simulink model "PruebaN5"  (R2024b)
settings: Solver=ode45  StartTime=0.0  StopTime=10  RelTol=1e-3
values from neighbouring files (symbols this model uses):
  T = 10e-3    (= 0.01)    [Proceso.m]    (also in regdiagSISOsep.m = Reg.Ts; regdiagsep.m = Reg.Ts; regsep.m = Reg.Ts)
undefined symbols (not defined in the file or in its folder): N, nl, nr, RegBal_Len2_ext, RegBal_Len3_ext, RegBal_Len4_ext, RegBal_Len5_ext, RegDiag_Len2_ext, RegDiag_Len3_ext, RegDiag_Len4_ext, RegDiag_Len5_ext, SR_Bal
libraries: cstblocks x18
settings Model: Creator=Guillem  LastModifiedBy=jroigro
settings SolverCC: AlgebraicLoopSolver=TrustRegion
settings DataIOCC: LimitDataPoints=on  SaveFormat=Array  SignalLoggingSaveFormat=ModelDataLogs  ReturnWorkspaceOutputs=off
settings OptimizationCC: BlockReduction=off  BooleanDataType=off  LifeSpan=inf
settings DebuggingCC: SaveWithParameterizedLinksMsg=none  UnderspecifiedInitializationDetection=Classic  MergeDetectMultiDrivingBlocksExec=none  SignalResolutionControl=TryResolveAllWithWarning  MultiTaskDSMMsg=warning  MultiTaskCondExecSysMsg=none  UnconnectedInputMsg=warning  UnconnectedOutputMsg=warning  UnconnectedLineMsg=warning  SFUnexpectedBacktrackingDiag=warning  SFNoUnconditionalDefaultTransitionDiag=warning  SFExecutionAtInitializationDiag=none  ArithmeticOperatorsInVariantConditions=warning
settings HardwareCC: ProdBitPerPointer=32  ProdBitPerSizeT=32  ProdBitPerPtrDiffT=32  ProdLargestAtomicFloat=None  ProdIntDivRoundTo=Undefined  ProdEndianess=Unspecified  ProdWordSize=32  ProdHWDeviceType=32-bit Generic  TargetUnknown=on
settings ModelReferenceCC: PropagateSignalLabelsOutOfModel=off
settings SFSimCC: SimUseLocalCustomCode=off  CustomCodeUndefinedFunction=UseInterfaceOnly
settings RTWCC: RTWUseLocalCustomCode=off  GPUComputeCapability=3.5
settings CodeAppCC: StateflowObjectComments=on
settings GRTTargetCC: TargetLangStandard=C89/C90 (ANSI)
settings ConfigComp: CovMetricSettings=dw  CovSaveCumulativeToWorkspaceVar=on  CovSaveSingleToWorkspaceVar=on  CovExternalEMLEnable=off

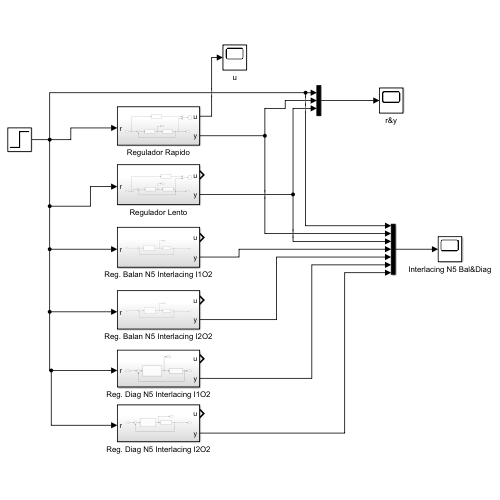
[thumbnail: Simulink's stored preview of the top-level diagram]
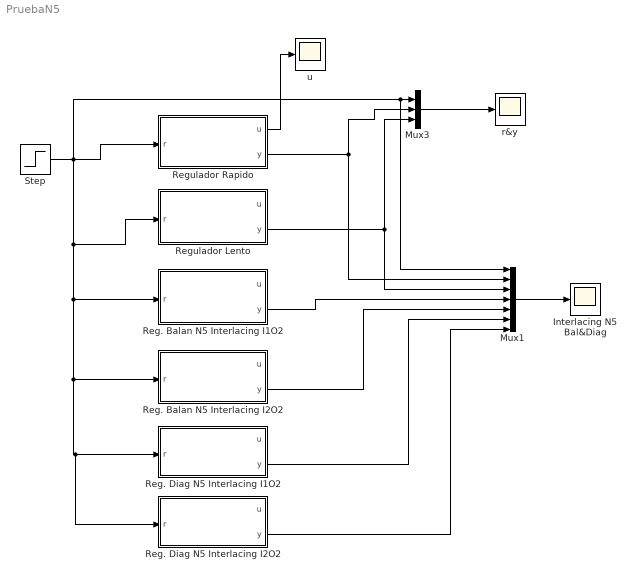
== system PruebaN5 ==
  Interlacing N5 Bal&Diag : Scope
  Mux1 : Mux  Inputs=7
  Mux3 : Mux  Inputs=3
  Reg. Balan N5 Interlacing I1O2 : Subsystem
  Reg. Balan N5 Interlacing I2O2 : Subsystem
  Reg. Diag N5 Interlacing I1O2 : Subsystem
  Reg. Diag N5 Interlacing I2O2 : Subsystem
  Regulador Lento : Subsystem
  Regulador Rapido : Subsystem
  Step : Step  Time=10  Before=1  After=2  SampleTime=0
  r&y : Scope
  u : Scope
  wires:
  Mux3/1 -> r&y/1
  Regulador Rapido/2(y) -> Mux1/2, Mux3/2
  Regulador Rapido/1(u) -> u/1
  Reg. Balan N5 Interlacing I2O2/2(y) -> Mux1/5
  Mux1/1 -> Interlacing N5 Bal&Diag/1
  Regulador Lento/2(y) -> Mux1/3, Mux3/3
  Reg. Balan N5 Interlacing I1O2/2(y) -> Mux1/4
  Step/1 -> Reg. Diag N5 Interlacing I2O2/1(r), Reg. Diag N5 Interlacing I1O2/1(r), Reg. Balan N5 Interlacing I2O2/1(r), Reg. Balan N5 Interlacing I1O2/1(r), Regulador Lento/1(r), Mux1/1, Mux3/1, Regulador Rapido/1(r)
  Reg. Diag N5 Interlacing I1O2/2(y) -> Mux1/6
  Reg. Diag N5 Interlacing I2O2/2(y) -> Mux1/7

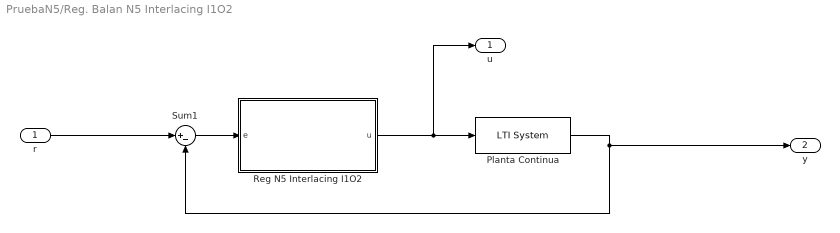
== system PruebaN5/Reg. Balan N5 Interlacing I1O2 ==
  r : Inport
  Planta Continua : cstblocks/LTI System  sys=Planta  IC=[]  PadeOrder=0
  Reg N5 Interlacing I1O2 : Subsystem
  Sum1 : Sum  Inputs=|+-
  u : Outport
  y : Outport  Port=2
  wires:
  Reg N5 Interlacing I1O2/1(u) -> u/1, Planta Continua/1
  Planta Continua/1 -> y/1, Sum1/2
  Sum1/1 -> Reg N5 Interlacing I1O2/1(e)
  r/1 -> Sum1/1

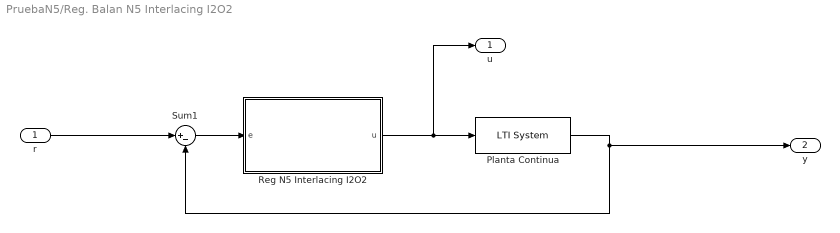
== system PruebaN5/Reg. Balan N5 Interlacing I2O2 ==
  r : Inport
  Planta Continua : cstblocks/LTI System  sys=Planta  IC=[]  PadeOrder=0
  Reg N5 Interlacing I2O2 : Subsystem
  Sum1 : Sum  Inputs=|+-
  u : Outport
  y : Outport  Port=2
  wires:
  r/1 -> Sum1/1
  Reg N5 Interlacing I2O2/1(u) -> u/1, Planta Continua/1
  Sum1/1 -> Reg N5 Interlacing I2O2/1(e)
  Planta Continua/1 -> y/1, Sum1/2

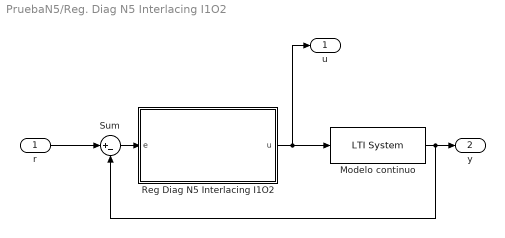
== system PruebaN5/Reg. Diag N5 Interlacing I1O2 ==
  r : Inport
  Modelo continuo : cstblocks/LTI System  sys=Planta  IC=[]  PadeOrder=0
  Reg Diag N5 Interlacing I1O2 : Subsystem
  Sum : Sum  Inputs=|+-
  u : Outport
  y : Outport  Port=2
  wires:
  Reg Diag N5 Interlacing I1O2/1(u) -> Modelo continuo/1, u/1
  r/1 -> Sum/1
  Sum/1 -> Reg Diag N5 Interlacing I1O2/1(e)
  Modelo continuo/1 -> Sum/2, y/1

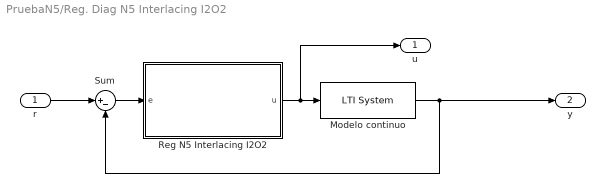
== system PruebaN5/Reg. Diag N5 Interlacing I2O2 ==
  r : Inport
  Modelo continuo : cstblocks/LTI System  sys=Planta  IC=[]  PadeOrder=0
  Reg N5 Interlacing I2O2 : Subsystem
  Sum : Sum  Inputs=|+-
  u : Outport
  y : Outport  Port=2
  wires:
  Modelo continuo/1 -> Sum/2, y/1
  Reg N5 Interlacing I2O2/1(u) -> Modelo continuo/1, u/1
  r/1 -> Sum/1
  Sum/1 -> Reg N5 Interlacing I2O2/1(e)

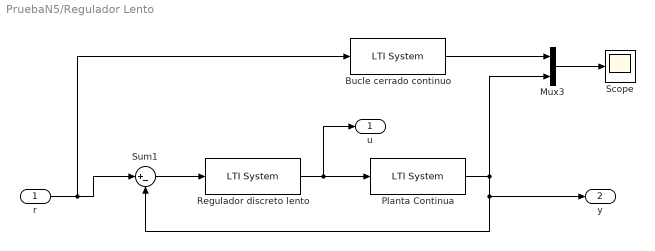
== system PruebaN5/Regulador Lento ==
  r : Inport
  Bucle cerrado continuo : cstblocks/LTI System  sys=BC2  IC=[]  PadeOrder=0
  Mux3 : Mux  Inputs=2
  Planta Continua : cstblocks/LTI System  sys=Planta  IC=[]  PadeOrder=0
  Regulador discreto lento : cstblocks/LTI System  sys=GrN5  IC=[]  PadeOrder=0
  Scope : Scope
  Sum1 : Sum  Inputs=|+-
  u : Outport
  y : Outport  Port=2
  wires:
  r/1 -> Bucle cerrado continuo/1, Sum1/1
  Regulador discreto lento/1 -> u/1, Planta Continua/1
  Sum1/1 -> Regulador discreto lento/1
  Planta Continua/1 -> Sum1/2, y/1, Mux3/2
  Mux3/1 -> Scope/1
  Bucle cerrado continuo/1 -> Mux3/1

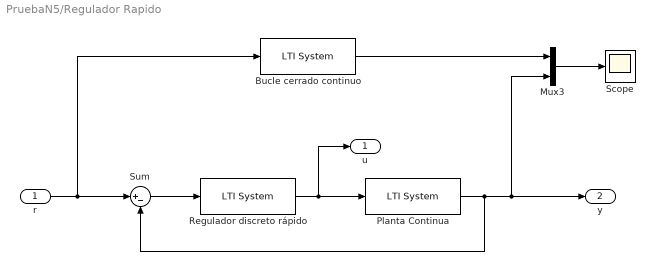
== system PruebaN5/Regulador Rapido ==
  r : Inport
  Bucle cerrado continuo : cstblocks/LTI System  sys=BC1  IC=[]  PadeOrder=0
  Mux3 : Mux  Inputs=2
  Planta Continua : cstblocks/LTI System  sys=Planta  IC=[]  PadeOrder=0
  Regulador discreto rápido : cstblocks/LTI System  sys=Gr  IC=[]  PadeOrder=0
  Scope : Scope
  Sum : Sum  Inputs=|+-
  u : Outport
  y : Outport  Port=2
  wires:
  Regulador discreto rápido/1 -> u/1, Planta Continua/1
  Bucle cerrado continuo/1 -> Mux3/1
  Mux3/1 -> Scope/1
  Sum/1 -> Regulador discreto rápido/1
  Planta Continua/1 -> Mux3/2, y/1, Sum/2
  r/1 -> Sum/1, Bucle cerrado continuo/1

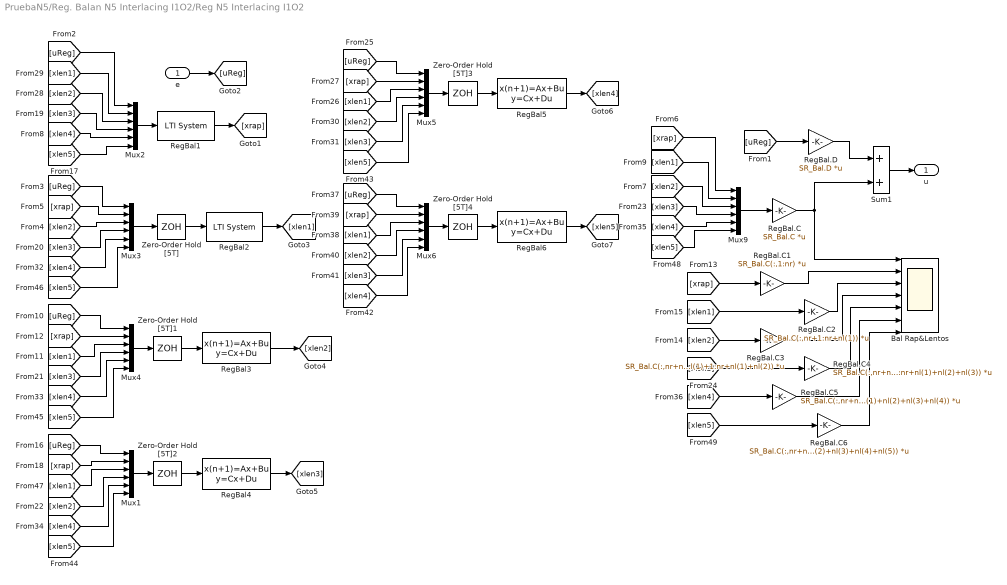
== system PruebaN5/Reg. Balan N5 Interlacing I1O2/Reg N5 Interlacing I1O2 ==
  e : Inport
  Bal Rap&Lentos : Scope  NumInputPorts=7
  Mux{1..6,9} (7 alike) : Mux  Inputs=6
  RegBal.C : Gain  Gain=SR_Bal.C  Multiplication=Matrix(K*u)
  RegBal.C1 : Gain  Gain=SR_Bal.C(:,1:nr)  Multiplication=Matrix(K*u)
  RegBal.C2 : Gain  Gain=SR_Bal.C(:,nr+1:nr+nl(1))  Multiplication=Matrix(K*u)
  RegBal.C3 : Gain  Gain=SR_Bal.C(:,nr+nl(1)+1:nr+nl(1)+nl(2))  Multiplication=Matrix(K*u)
  RegBal.C4 : Gain  Gain=SR_Bal.C(:,nr+nl(1)+nl(2)+1:nr+nl(1)+nl(2)+nl(3))  Multiplication=Matrix(K*u)
  RegBal.C5 : Gain  Gain=SR_Bal.C(:,nr+nl(1)+nl(2)+nl(3)+1:nr+nl(1)+nl(2)+nl(3)+nl(4))  Multiplication=Matrix(K*u)
  RegBal.C6 : Gain  Gain=SR_Bal.C(:,nr+nl(1)+nl(2)+nl(3)+nl(4)+1:nr+nl(1)+nl(2)+nl(3)+nl(4)+nl(5))  Multiplication=Matrix(K*u)
  RegBal.D : Gain  Gain=SR_Bal.D  Multiplication=Matrix(K*u)
  RegBal1 : cstblocks/LTI System  sys=RegBal_Rap  IC=[]  PadeOrder=0
  RegBal2 : cstblocks/LTI System  sys=RegBal_Len1_ext  IC=[]  PadeOrder=0
  RegBal3 : DiscreteStateSpace  A=RegBal_Len2_ext.A  B=RegBal_Len2_ext.B  C=RegBal_Len2_ext.C  D=RegBal_Len2_ext.D  SampleTime=[N*T,T]
  RegBal4 : DiscreteStateSpace  A=RegBal_Len3_ext.A  B=RegBal_Len3_ext.B  C=RegBal_Len3_ext.C  D=RegBal_Len3_ext.D  SampleTime=[N*T,2*T]
  RegBal5 : DiscreteStateSpace  A=RegBal_Len4_ext.A  B=RegBal_Len4_ext.B  C=RegBal_Len4_ext.C  D=RegBal_Len4_ext.D  SampleTime=[N*T,3*T]
  RegBal6 : DiscreteStateSpace  A=RegBal_Len5_ext.A  B=RegBal_Len5_ext.B  C=RegBal_Len5_ext.C  D=RegBal_Len5_ext.D  SampleTime=[N*T,4*T]
  Sum1 : Sum
  Zero-Order Hold [5T]{,1..4} (5 alike) : ZeroOrderHold  SampleTime=[N*T]
  u : Outport
  wires:
  RegBal.D/1 -> Sum1/1
  Mux4/1 -> Zero-Order Hold [5T]1/1
  Mux9/1 -> RegBal.C/1
  Sum1/1 -> u/1
  Mux2/1 -> RegBal1/1
  Mux3/1 -> Zero-Order Hold [5T]/1
  e/1 -> [uReg]
  RegBal.C3/1 -> Bal Rap&Lentos/4
  RegBal.C/1 -> Bal Rap&Lentos/1, Sum1/2
  RegBal.C2/1 -> Bal Rap&Lentos/3
  RegBal2/1 -> [xlen1]
  RegBal.C1/1 -> Bal Rap&Lentos/2
  Zero-Order Hold [5T]/1 -> RegBal2/1
  Zero-Order Hold [5T]1/1 -> RegBal3/1
  RegBal1/1 -> [xrap]
  [uReg] -> RegBal.D/1
  [uReg] -> Mux2/1
  [xlen1] -> Mux2/2
  [xlen2] -> Mux2/3
  [uReg] -> Mux3/1
  [xlen2] -> Mux3/3
  [xrap] -> Mux3/2
  [xrap] -> Mux9/1
  [xlen1] -> Mux9/2
  [xlen2] -> Mux9/3
  RegBal3/1 -> [xlen2]
  [xrap] -> Mux4/2
  [xlen1] -> Mux4/3
  [uReg] -> Mux4/1
  [xlen2] -> RegBal.C3/1
  [xlen1] -> RegBal.C2/1
  [xrap] -> RegBal.C1/1
  [uReg] -> Mux1/1
  [xrap] -> Mux1/2
  RegBal4/1 -> [xlen3]
  Zero-Order Hold [5T]2/1 -> RegBal4/1
  Mux1/1 -> Zero-Order Hold [5T]2/1
  [xlen3] -> Mux2/4
  [xlen3] -> Mux3/4
  [xlen3] -> Mux4/4
  [xlen2] -> Mux1/4
  [xlen3] -> Mux9/4
  [xlen3] -> RegBal.C4/1
  RegBal.C4/1 -> Bal Rap&Lentos/5
  [xlen1] -> Mux5/3
  Zero-Order Hold [5T]3/1 -> RegBal5/1
  [xrap] -> Mux5/2
  [uReg] -> Mux5/1
  Mux5/1 -> Zero-Order Hold [5T]3/1
  [xlen2] -> Mux5/4
  RegBal5/1 -> [xlen4]
  [xlen3] -> Mux5/5
  [xlen4] -> Mux2/5
  [xlen4] -> Mux3/5
  [xlen4] -> Mux4/5
  [xlen4] -> Mux1/5
  [xlen4] -> Mux9/5
  [xlen4] -> RegBal.C5/1
  RegBal.C5/1 -> Bal Rap&Lentos/6
  [xlen3] -> Mux6/5
  RegBal6/1 -> [xlen5]
  [xlen2] -> Mux6/4
  Mux6/1 -> Zero-Order Hold [5T]4/1
  [uReg] -> Mux6/1
  [xrap] -> Mux6/2
  Zero-Order Hold [5T]4/1 -> RegBal6/1
  [xlen1] -> Mux6/3
  [xlen4] -> Mux6/6
  [xlen5] -> Mux5/6
  [xlen5] -> Mux1/6
  [xlen5] -> Mux4/6
  [xlen5] -> Mux3/6
  [xlen1] -> Mux1/3
  [xlen5] -> Mux2/6
  [xlen5] -> Mux9/6
  [xlen5] -> RegBal.C6/1
  RegBal.C6/1 -> Bal Rap&Lentos/7

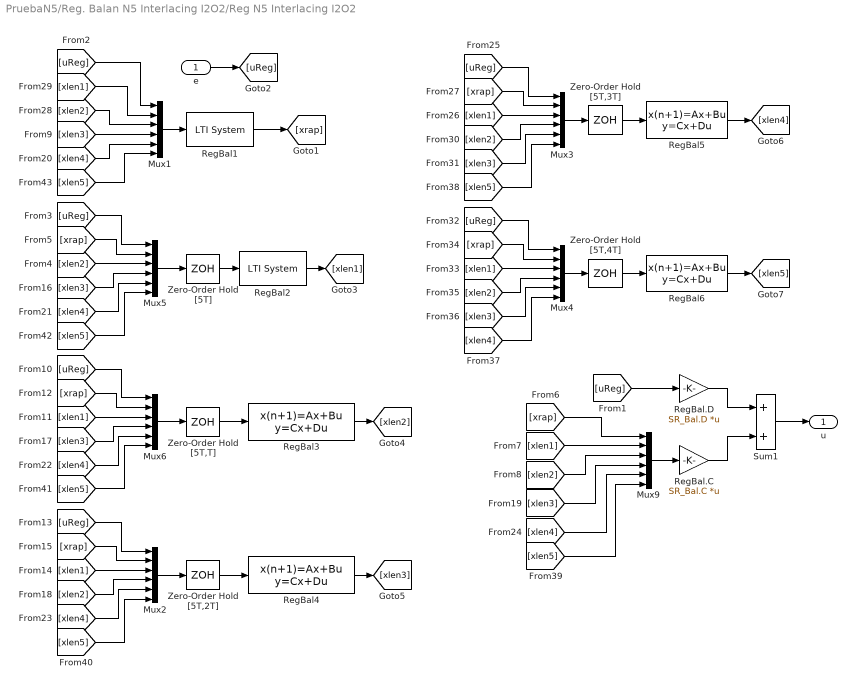
== system PruebaN5/Reg. Balan N5 Interlacing I2O2/Reg N5 Interlacing I2O2 ==
  e : Inport
  Mux{1..6,9} (7 alike) : Mux  Inputs=6
  RegBal.C : Gain  Gain=SR_Bal.C  Multiplication=Matrix(K*u)
  RegBal.D : Gain  Gain=SR_Bal.D  Multiplication=Matrix(K*u)
  RegBal1 : cstblocks/LTI System  sys=RegBal_Rap  IC=[]  PadeOrder=0
  RegBal2 : cstblocks/LTI System  sys=RegBal_Len1_ext  IC=[]  PadeOrder=0
  RegBal3 : DiscreteStateSpace  A=RegBal_Len2_ext.A  B=RegBal_Len2_ext.B  C=RegBal_Len2_ext.C  D=RegBal_Len2_ext.D  SampleTime=[N*T,T]
  RegBal4 : DiscreteStateSpace  A=RegBal_Len3_ext.A  B=RegBal_Len3_ext.B  C=RegBal_Len3_ext.C  D=RegBal_Len3_ext.D  SampleTime=[N*T,2*T]
  RegBal5 : DiscreteStateSpace  A=RegBal_Len4_ext.A  B=RegBal_Len4_ext.B  C=RegBal_Len4_ext.C  D=RegBal_Len4_ext.D  SampleTime=[N*T,3*T]
  RegBal6 : DiscreteStateSpace  A=RegBal_Len5_ext.A  B=RegBal_Len5_ext.B  C=RegBal_Len5_ext.C  D=RegBal_Len5_ext.D  SampleTime=[N*T,4*T]
  Sum1 : Sum
  Zero-Order Hold [5T,2T] : ZeroOrderHold  SampleTime=[N*T,2*T]
  Zero-Order Hold [5T,3T] : ZeroOrderHold  SampleTime=[N*T,3*T]
  Zero-Order Hold [5T,4T] : ZeroOrderHold  SampleTime=[N*T,4*T]
  Zero-Order Hold [5T,T] : ZeroOrderHold  SampleTime=[N*T,T]
  Zero-Order Hold [5T] : ZeroOrderHold  SampleTime=[N*T]
  u : Outport
  wires:
  RegBal.C/1 -> Sum1/2
  Sum1/1 -> u/1
  Mux9/1 -> RegBal.C/1
  Mux6/1 -> Zero-Order Hold [5T,T]/1
  RegBal.D/1 -> Sum1/1
  Zero-Order Hold [5T,T]/1 -> RegBal3/1
  Zero-Order Hold [5T]/1 -> RegBal2/1
  [xlen1] -> Mux1/2
  [xrap] -> Mux5/2
  e/1 -> [uReg]
  Mux5/1 -> Zero-Order Hold [5T]/1
  [xlen2] -> Mux1/3
  [xlen2] -> Mux5/3
  [uReg] -> Mux5/1
  [xrap] -> Mux6/2
  [xlen1] -> Mux6/3
  [uReg] -> Mux6/1
  [uReg] -> Mux1/1
  Mux1/1 -> RegBal1/1
  RegBal1/1 -> [xrap]
  RegBal2/1 -> [xlen1]
  RegBal3/1 -> [xlen2]
  [uReg] -> RegBal.D/1
  [xrap] -> Mux9/1
  [xlen1] -> Mux9/2
  [xlen2] -> Mux9/3
  RegBal4/1 -> [xlen3]
  [uReg] -> Mux2/1
  [xlen1] -> Mux2/3
  [xrap] -> Mux2/2
  Zero-Order Hold [5T,2T]/1 -> RegBal4/1
  Mux2/1 -> Zero-Order Hold [5T,2T]/1
  [xlen3] -> Mux1/4
  [xlen3] -> Mux5/4
  [xlen3] -> Mux6/4
  [xlen2] -> Mux2/4
  [xlen3] -> Mux9/4
  RegBal5/1 -> [xlen4]
  Mux3/1 -> Zero-Order Hold [5T,3T]/1
  [xlen2] -> Mux3/4
  [uReg] -> Mux3/1
  [xrap] -> Mux3/2
  [xlen3] -> Mux3/5
  Zero-Order Hold [5T,3T]/1 -> RegBal5/1
  [xlen1] -> Mux3/3
  [xlen4] -> Mux1/5
  [xlen4] -> Mux5/5
  [xlen4] -> Mux6/5
  [xlen4] -> Mux2/5
  [xlen4] -> Mux9/5
  [uReg] -> Mux4/1
  Zero-Order Hold [5T,4T]/1 -> RegBal6/1
  Mux4/1 -> Zero-Order Hold [5T,4T]/1
  RegBal6/1 -> [xlen5]
  [xlen2] -> Mux4/4
  [xlen3] -> Mux4/5
  [xlen1] -> Mux4/3
  [xrap] -> Mux4/2
  [xlen4] -> Mux4/6
  [xlen5] -> Mux3/6
  [xlen5] -> Mux9/6
  [xlen5] -> Mux2/6
  [xlen5] -> Mux6/6
  [xlen5] -> Mux5/6
  [xlen5] -> Mux1/6

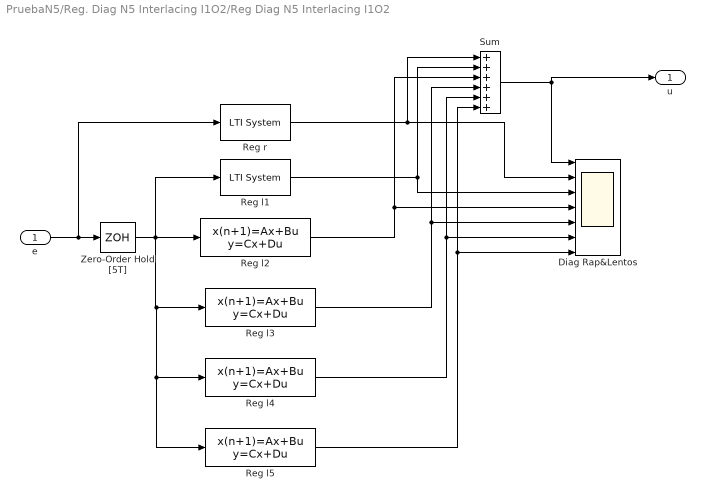
== system PruebaN5/Reg. Diag N5 Interlacing I1O2/Reg Diag N5 Interlacing I1O2 ==
  e : Inport
  Diag Rap&Lentos : Scope  NumInputPorts=7
  Reg l1 : cstblocks/LTI System  sys=RegDiag_Len1_ext  IC=[]  PadeOrder=0
  Reg l2 : DiscreteStateSpace  A=RegDiag_Len2_ext.A  B=RegDiag_Len2_ext.B  C=RegDiag_Len2_ext.C  D=RegDiag_Len2_ext.D  SampleTime=[N*T,T]
  Reg l3 : DiscreteStateSpace  A=RegDiag_Len3_ext.A  B=RegDiag_Len3_ext.B  C=RegDiag_Len3_ext.C  D=RegDiag_Len3_ext.D  SampleTime=[N*T,2*T]
  Reg l4 : DiscreteStateSpace  A=RegDiag_Len4_ext.A  B=RegDiag_Len4_ext.B  C=RegDiag_Len4_ext.C  D=RegDiag_Len4_ext.D  SampleTime=[N*T,3*T]
  Reg l5 : DiscreteStateSpace  A=RegDiag_Len5_ext.A  B=RegDiag_Len5_ext.B  C=RegDiag_Len5_ext.C  D=RegDiag_Len5_ext.D  SampleTime=[N*T,4*T]
  Reg r : cstblocks/LTI System  sys=RegDiag_Rap  IC=[]  PadeOrder=0
  Sum : Sum  Inputs=++++++
  Zero-Order Hold [5T] : ZeroOrderHold  SampleTime=[N*T]
  u : Outport
  wires:
  Sum/1 -> u/1, Diag Rap&Lentos/1
  Reg l1/1 -> Diag Rap&Lentos/3, Sum/2
  Reg r/1 -> Sum/1, Diag Rap&Lentos/2
  e/1 -> Reg r/1, Zero-Order Hold [5T]/1
  Zero-Order Hold [5T]/1 -> Reg l5/1, Reg l4/1, Reg l3/1, Reg l1/1, Reg l2/1
  Reg l2/1 -> Sum/3, Diag Rap&Lentos/4
  Reg l3/1 -> Diag Rap&Lentos/5, Sum/4
  Reg l4/1 -> Diag Rap&Lentos/6, Sum/5
  Reg l5/1 -> Diag Rap&Lentos/7, Sum/6

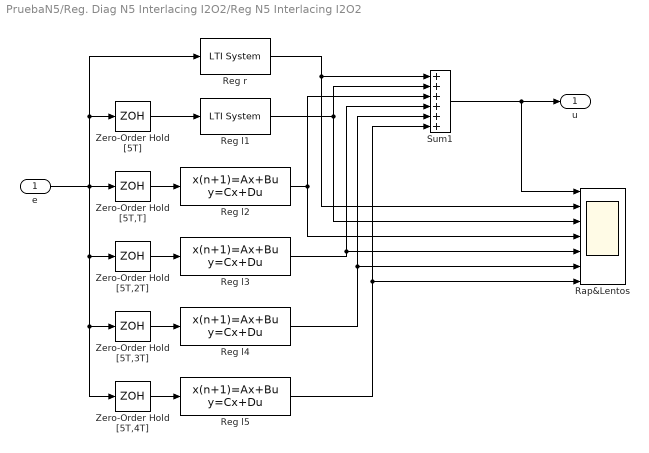
== system PruebaN5/Reg. Diag N5 Interlacing I2O2/Reg N5 Interlacing I2O2 ==
  e : Inport
  Rap&Lentos : Scope  NumInputPorts=7
  Reg l1 : cstblocks/LTI System  sys=RegDiag_Len1_ext  IC=[]  PadeOrder=0
  Reg l2 : DiscreteStateSpace  A=RegDiag_Len2_ext.A  B=RegDiag_Len2_ext.B  C=RegDiag_Len2_ext.C  D=RegDiag_Len2_ext.D  SampleTime=[N*T,T]
  Reg l3 : DiscreteStateSpace  A=RegDiag_Len3_ext.A  B=RegDiag_Len3_ext.B  C=RegDiag_Len3_ext.C  D=RegDiag_Len3_ext.D  SampleTime=[N*T,2*T]
  Reg l4 : DiscreteStateSpace  A=RegDiag_Len4_ext.A  B=RegDiag_Len4_ext.B  C=RegDiag_Len4_ext.C  D=RegDiag_Len4_ext.D  SampleTime=[N*T,3*T]
  Reg l5 : DiscreteStateSpace  A=RegDiag_Len5_ext.A  B=RegDiag_Len5_ext.B  C=RegDiag_Len5_ext.C  D=RegDiag_Len5_ext.D  SampleTime=[N*T,4*T]
  Reg r : cstblocks/LTI System  sys=RegDiag_Rap  IC=[]  PadeOrder=0
  Sum1 : Sum  Inputs=++++++
  Zero-Order Hold [5T,2T] : ZeroOrderHold  SampleTime=[N*T,2*T]
  Zero-Order Hold [5T,3T] : ZeroOrderHold  SampleTime=[N*T,3*T]
  Zero-Order Hold [5T,4T] : ZeroOrderHold  SampleTime=[N*T,4*T]
  Zero-Order Hold [5T,T] : ZeroOrderHold  SampleTime=[N*T,T]
  Zero-Order Hold [5T] : ZeroOrderHold  SampleTime=[N*T]
  u : Outport
  wires:
  Reg l2/1 -> Rap&Lentos/4, Sum1/3
  Reg r/1 -> Rap&Lentos/2, Sum1/1
  Reg l1/1 -> Rap&Lentos/3, Sum1/2
  Sum1/1 -> u/1, Rap&Lentos/1
  Zero-Order Hold [5T,T]/1 -> Reg l2/1
  Zero-Order Hold [5T]/1 -> Reg l1/1
  Zero-Order Hold [5T,2T]/1 -> Reg l3/1
  Reg l3/1 -> Sum1/4, Rap&Lentos/5
  Zero-Order Hold [5T,3T]/1 -> Reg l4/1
  e/1 -> Zero-Order Hold [5T,4T]/1, Zero-Order Hold [5T,3T]/1, Zero-Order Hold [5T,2T]/1, Zero-Order Hold [5T,T]/1, Zero-Order Hold [5T]/1, Reg r/1
  Reg l4/1 -> Rap&Lentos/6, Sum1/5
  Zero-Order Hold [5T,4T]/1 -> Reg l5/1
  Reg l5/1 -> Rap&Lentos/7, Sum1/6
